simulink model "CC"  (R2021b)
settings: Solver=ode8  StartTime=0.0  StopTime=60  FixedStep=0.01  RelTol=1e-3
values from neighbouring files (symbols this model uses):
  b = 50    [CC_PID.mat]
  m = 1000    [CC_PID.mat]
settings Model: Creator=Manmath Kharade  LastModifiedBy=Manmath Kharade
settings OptimizationCC: DefaultParameterBehavior=Inlined  GainParamInheritBuiltInType=on  UseFloatMulNetSlope=on  InlineInvariantSignals=on  EfficientFloat2IntCast=on
settings DebuggingCC: AlgebraicLoopMsg=none
settings RTWCC: GenerateReport=on  BuildConfiguration=Faster Runs  LaunchReport=on
settings CodeAppCC: ForceParamTrailComments=on  MATLABSourceComments=on
settings GRTTargetCC: MatFileLogging=off  SupportNonFinite=off

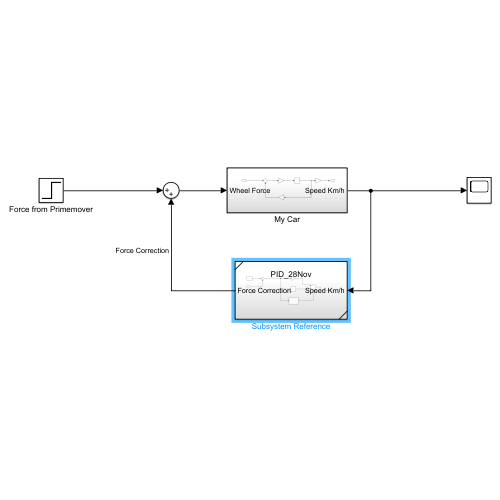
[thumbnail: Simulink's stored preview of the top-level diagram]
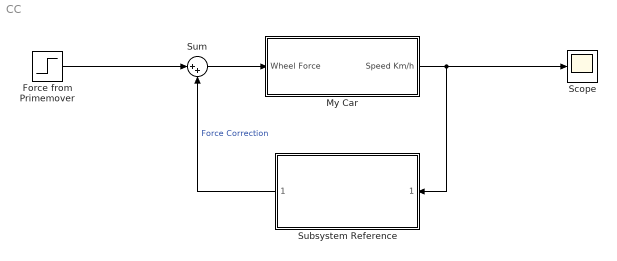
== system CC ==
  Force from Primemover : Step  Time=0  After=u  SampleTime=0.01
  My Car : Subsystem
  Scope : Scope
  Subsystem Reference : Subsystem  ReferencedSubsystem=PID_28Nov
  Sum : Sum  Inputs=|++
  wires:
  Subsystem Reference/1 -> Sum/2  "Force Correction"
  Force from Primemover/1 -> Sum/1
  My Car/1(Speed Km/h) -> Scope/1, Subsystem Reference/1
  Sum/1 -> My Car/1(Wheel Force)

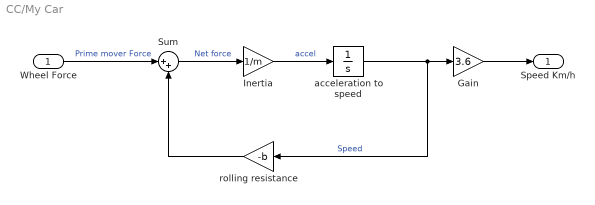
== system CC/My Car ==
  Wheel Force : Inport
  Gain : Gain  Gain=3.6
  Inertia : Gain  Gain=1/m
  Sum : Sum  Inputs=|++
  acceleration to speed : Integrator
  rolling resistance : Gain  Gain=-b
  Speed Km/h : Outport
  wires:
  acceleration to speed/1 -> Gain/1, rolling resistance/1  "Speed"
  Sum/1 -> Inertia/1  "Net force"
  Wheel Force/1 -> Sum/1  "Prime mover Force"
  rolling resistance/1 -> Sum/2
  Inertia/1 -> acceleration to speed/1  "accel"
  Gain/1 -> Speed Km/h/1
